simulink model "OVERALL_robust"  (R2021a)
settings: Solver=ode45  StartTime=0.0  StopTime=20  MaxStep=0.001  RelTol=1e-3
values from neighbouring files (symbols this model uses):
  disturbance = 5/drv.duty2V    [SSController_nominal.m]    (also in SSController_robust.m)
  ref = 0.1/wheel.r    [SSController_nominal.m]    (also in SSController_robust.m)
  Ts = 0.01    [SSController_nominal.m]    (also in SSController_robust.m; balancing_robot_params.m)
settings Model: Creator=umberto  LastModifiedBy=utente-A
settings SolverCC: AlgebraicLoopSolver=TrustRegion
settings DebuggingCC: SFMachineParentedDataDiag=warning

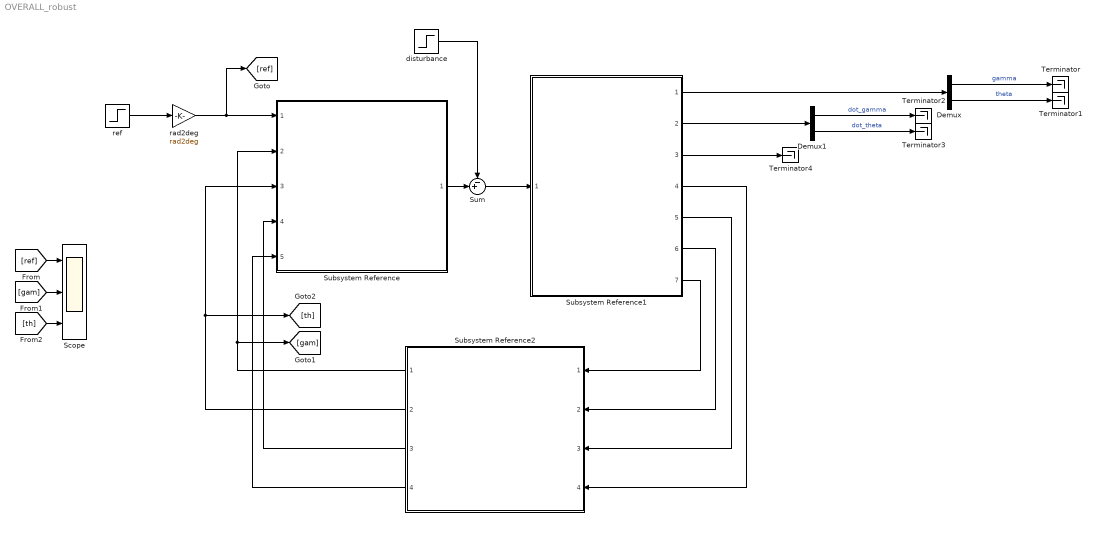
== system OVERALL_robust ==
  Demux : Demux  Outputs=2
  Demux1 : Demux  Outputs=2
  Scope : Scope  NumInputPorts=3
  Subsystem Reference : Subsystem  ReferencedSubsystem=StateSpaceControllerRobust_SubSystem
  Subsystem Reference1 : Subsystem  ReferencedSubsystem=balrobot_SubSystem
  Subsystem Reference2 : Subsystem  ReferencedSubsystem=SimpleStateObserver_SubSystem
  Sum : Sum  Inputs=-+|
  Terminator{,1..4} (5 alike) : Terminator
  disturbance : Step  Time=10  After=disturbance  SampleTime=Ts
  rad2deg : Gain  Gain=rad2deg
  ref : Step  Time=0  After=ref  SampleTime=Ts
  wires:
  Subsystem Reference2/1 -> Subsystem Reference/2, [gam]
  Subsystem Reference2/2 -> Subsystem Reference/3, [th]
  Subsystem Reference2/3 -> Subsystem Reference/4
  Subsystem Reference2/4 -> Subsystem Reference/5
  Demux/2 -> Terminator1/1  "theta"
  Demux/1 -> Terminator/1  "gamma"
  rad2deg/1 -> Subsystem Reference/1, [ref]
  Subsystem Reference/1 -> Sum/2
  Sum/1 -> Subsystem Reference1/1
  Subsystem Reference1/1 -> Demux/1
  Subsystem Reference1/2 -> Demux1/1
  Demux1/2 -> Terminator3/1  "dot_theta"
  Demux1/1 -> Terminator2/1  "dot_gamma"
  Subsystem Reference1/3 -> Terminator4/1
  Subsystem Reference1/7 -> Subsystem Reference2/1
  Subsystem Reference1/6 -> Subsystem Reference2/2
  Subsystem Reference1/5 -> Subsystem Reference2/3
  Subsystem Reference1/4 -> Subsystem Reference2/4
  disturbance/1 -> Sum/1
  ref/1 -> rad2deg/1
  [gam] -> Scope/2
  [ref] -> Scope/1
  [th] -> Scope/3
